simulink model "Assignment2"  (R2020a)
settings: Solver=FixedStepAuto  StartTime=0.0  StopTime=10.0  FixedStep=1e-3  RelTol=1e-3  EnableMultiTasking=on
undefined symbols (not defined in the file or in its folder): D0, D1, D10, D11, D12, D13, D2, D3, D4, D5, D6, D7, D8, D9, PTA0, PTA1, PTA2, PTB23, PTB9, PTC16, PTC17, PTC2, PTC3, PTC4, PTD0, PTD1, PTD2, PTD3
libraries: frdmk64flib x18, etargetslib x5
settings Model: ExtModeTrigDuration=5  Creator=iceca  LastModifiedBy=iceca
settings OptimizationCC: EnhancedBackFolding=on  PassReuseOutputArgsAs=Individual arguments  ZeroExternalMemoryAtStartup=off  ZeroInternalMemoryAtStartup=off  MaxStackSize=64  OptimizeBlockOrder=speed  DifferentSizesBufferReuse=on  OptimizationCustomize=off  EfficientTunableParamExpr=on
settings DebuggingCC: ParameterTunabilityLossMsg=error
settings HardwareCC: ProdBitPerPointer=32  ProdBitPerSizeT=32  ProdBitPerPtrDiffT=32  ProdLargestAtomicInteger=Long  ProdLargestAtomicFloat=Double  ProdWordSize=32  ProdHWDeviceType=ARM Compatible->ARM Cortex
settings SFSimCC: MATLABDynamicMemAlloc=off
settings RTWCC: SystemTargetFile=ert.tlc  HardwareBoard=NXP FRDM-K64F  TemplateMakefile=ert_default_tmf  Toolchain=GNU Tools for ARM Embedded Processors
settings CodeAppCC: ForceParamTrailComments=on  IgnoreCustomStorageClasses=off  OperatorAnnotations=on  SimulinkDataObjDesc=on  SFDataObjDesc=on  InsertBlockDesc=on

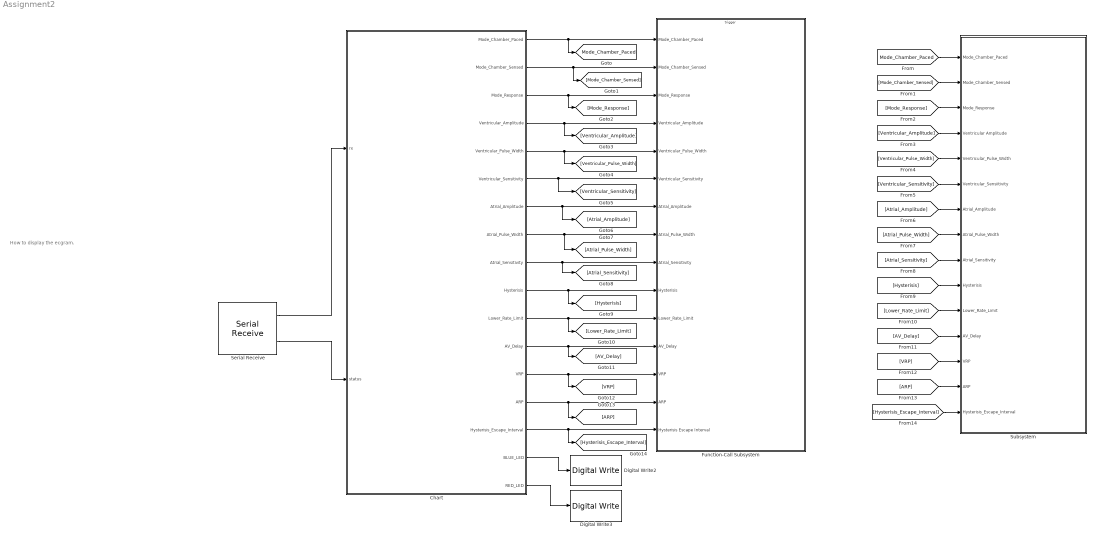
== system Assignment2 ==
  note: How to display the ecgram.
  Chart : Stateflow chart  TreatAsAtomicUnit=on
  Digital Write2 : frdmk64flib/Digital Write  Whichpin=BLUE_LED
  Digital Write3 : frdmk64flib/Digital Write  Whichpin=RED_LED
  Function-Call Subsystem : Subsystem  TreatAsAtomicUnit=on
  Serial Receive : frdmk64flib/Serial Receive  SCIModule=0  Baudrate=uint32(9600)  Parity=None  StopBits=1  HardwareFlowControl=None  ByteOrder=LittleEndian  DataType=uint8  DataLength=22  BlockingMode=off  OutputStatus=on  SampleTime=-1
  Subsystem : Subsystem
  tag scope: Mode_Chamber_Paced=global
  wires:
  Serial Receive/1 -> Chart/1(rx)
  Serial Receive/2 -> Chart/2(status)
  Chart/16(BLUE_LED) -> Digital Write2/1
  Chart/17(RED_LED) -> Digital Write3/1
  Chart/1(Mode_Chamber_Paced) -> [Mode_Chamber_Paced], Function-Call Subsystem/1(Mode_Chamber_Paced)
  Chart/10(Hysterisis) -> [Hysterisis], Function-Call Subsystem/10(Hysterisis)
  Chart/11(Lower_Rate_Limit) -> [Lower_Rate_Limit], Function-Call Subsystem/11(Lower_Rate_Limit)
  Chart/12(AV_Delay) -> [AV_Delay], Function-Call Subsystem/12(AV_Delay)
  Chart/13(VRP) -> [VRP], Function-Call Subsystem/13(VRP)
  Chart/14(ARP) -> [ARP], Function-Call Subsystem/14(ARP)
  Chart/15(Hysterisis_Escape_Interval) -> [Hysterisis_Escape_Interval], Function-Call Subsystem/15(Hysterisis Escape Interval)
  [Mode_Chamber_Paced] -> Subsystem/1(Mode_Chamber_Paced)
  Chart/2(Mode_Chamber_Sensed) -> [Mode_Chamber_Sensed], Function-Call Subsystem/2(Mode_Chamber_Sensed)
  Chart/3(Mode_Response) -> [Mode_Response], Function-Call Subsystem/3(Mode_Response)
  Chart/4(Ventricular_Amplitude) -> [Ventricular_Amplitude], Function-Call Subsystem/4(Ventricular_Amplitude)
  Chart/5(Ventricular_Pulse_Width) -> [Ventricular_Pulse_Width], Function-Call Subsystem/5(Ventricular_Pulse_Width)
  Chart/6(Ventricular_Sensitivity) -> [Ventricular_Sensitivity], Function-Call Subsystem/6(Ventricular_Sensitivity)
  Chart/7(Atrial_Amplitude) -> [Atrial_Amplitude], Function-Call Subsystem/7(Atrial_Amplitude)
  Chart/8(Atrial_Pulse_Width) -> [Atrial_Pulse_Width], Function-Call Subsystem/8(Atrial_Pulse_Width)
  Chart/9(Atrial_Sensitivity) -> [Atrial_Sensitivity], Function-Call Subsystem/9(Atrial_Sensitivity)
  [Mode_Chamber_Sensed] -> Subsystem/2(Mode_Chamber_Sensed)
  [Mode_Response] -> Subsystem/3(Mode_Response)
  [Ventricular_Amplitude] -> Subsystem/4(Ventricular Amplitude)
  [Ventricular_Pulse_Width] -> Subsystem/5(Ventricular_Pulse_Width)
  [Ventricular_Sensitivity] -> Subsystem/6(Ventricular_Sensiitivity)
  [Atrial_Amplitude] -> Subsystem/7(Atrial_Amplitude)
  [Atrial_Pulse_Width] -> Subsystem/8(Atrial_Pulse_Width)
  [Atrial_Sensitivity] -> Subsystem/9(Atrial_Sensitivity)
  [Hysterisis] -> Subsystem/10(Hysterisis)
  [Lower_Rate_Limit] -> Subsystem/11(Lower_Rate_Limit)
  [AV_Delay] -> Subsystem/12(AV_Delay)
  [VRP] -> Subsystem/13(VRP)
  [ARP] -> Subsystem/14(ARP)
  [Hysterisis_Escape_Interval] -> Subsystem/15(Hysterisis_Escape_Interval)

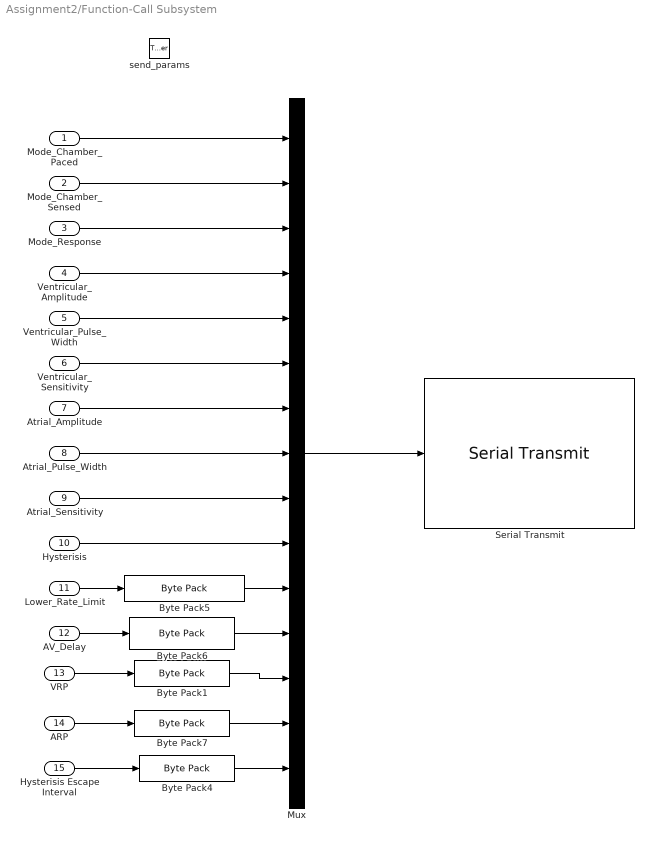
== system Assignment2/Function-Call Subsystem ==
  Mode_Chamber_Paced : Inport
  Mode_Chamber_Sensed : Inport  Port=2
  Mode_Response : Inport  Port=3
  Ventricular_Amplitude : Inport  Port=4
  Ventricular_Pulse_Width : Inport  Port=5
  Ventricular_Sensitivity : Inport  Port=6
  Atrial_Amplitude : Inport  Port=7
  Atrial_Pulse_Width : Inport  Port=8
  Atrial_Sensitivity : Inport  Port=9
  Hysterisis : Inport  Port=10
  Lower_Rate_Limit : Inport  Port=11
  AV_Delay : Inport  Port=12
  VRP : Inport  Port=13
  ARP : Inport  Port=14
  Hysterisis Escape Interval : Inport  Port=15
  send_params : TriggerPort  TriggerType=function-call  IsSimulinkFunction=on  FunctionName=send_params  VariantControl=Variant
  Byte Pack{1,4..7} (5 alike) : etargetslib/Byte Pack  datatypes={'uint16'}  byteAlign=1
  Mux : Mux  Inputs=15
  Serial Transmit : frdmk64flib/Serial Transmit  SCIModule=0  Baudrate=uint32(9600)  Parity=None  StopBits=1  HardwareFlowControl=None  ByteOrder=LittleEndian  BlockingMode=on  OutputStatus=off
  wires:
  Mode_Chamber_Paced/1 -> Mux/1
  Hysterisis/1 -> Mux/10
  Atrial_Pulse_Width/1 -> Mux/8
  Atrial_Amplitude/1 -> Mux/7
  Ventricular_Sensitivity/1 -> Mux/6
  Mode_Response/1 -> Mux/3
  Mode_Chamber_Sensed/1 -> Mux/2
  Atrial_Sensitivity/1 -> Mux/9
  Byte Pack1/1 -> Mux/13
  VRP/1 -> Byte Pack1/1
  Mux/1 -> Serial Transmit/1
  Ventricular_Amplitude/1 -> Mux/4
  Ventricular_Pulse_Width/1 -> Mux/5
  Hysterisis Escape Interval/1 -> Byte Pack4/1
  Lower_Rate_Limit/1 -> Byte Pack5/1
  AV_Delay/1 -> Byte Pack6/1
  Byte Pack6/1 -> Mux/12
  Byte Pack5/1 -> Mux/11
  Byte Pack7/1 -> Mux/14
  Byte Pack4/1 -> Mux/15
  ARP/1 -> Byte Pack7/1

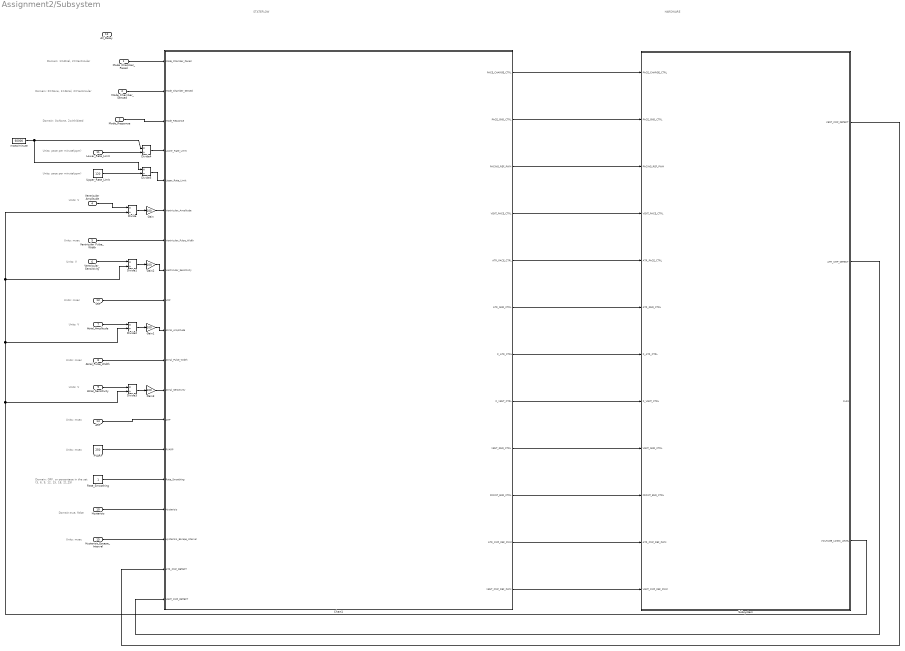
== system Assignment2/Subsystem ==
  note: Domain: OFF, or percentage
      | in the set (3, 6, 9, 12, 15, 18, 21,25)
  note: Domain: 0=None, 2=Inhibited
  note: Domain: 1=Atrial, 2=Ventricular
  note: Units: msec
  note: Units: pace per minute(ppm)
  note: HARDWARE
  note: Units: V
  note: STATEFLOW
  note: Units: msec
  note: Units: V
  note: Domain: 0=None, 1=Atrial, 2=Ventricular
  note: Units: pace per minute(ppm)
  note: Units: msec
  note: Units: msec
  note: Domain:true, false
  note: Units: V
  note: Units: msec
  note: Units: msec
  note: Units: V
  Mode_Chamber_Paced : Inport
  Mode_Chamber_Sensed : Inport  Port=2
  Mode_Response : Inport  Port=3
  Ventricular Amplitude : Inport  Port=4
  Ventricular_Pulse_Width : Inport  Port=5
  Ventricular_Sensiitivity : Inport  Port=6
  Atrial_Amplitude : Inport  Port=7
  Atrial_Pulse_Width : Inport  Port=8
  Atrial_Sensitivity : Inport  Port=9
  Hysterisis : Inport  Port=10
  Lower_Rate_Limit : Inport  Port=11
  AV_Delay : Inport  Port=12
  VRP : Inport  Port=13
  ARP : Inport  Port=14
  Hysterisis_Escape_Interval : Inport  Port=15
  Chart1 : Stateflow chart  TreatAsAtomicUnit=on
  Divide{,1..5} (6 alike) : Product  Inputs=*/
  Gain{,1..3} (4 alike) : Gain  Gain=100
  PVARP : Constant  Value=250
  Rate_Smoothing : Constant
  Subsystem : Subsystem
  Upper_Rate_Limit : Constant  Value=120
  msec/minute : Constant  Value=60000
  wires:
  Divide4/1 -> Chart1/4(Lower_Rate_Limit)
  Atrial_Pulse_Width/1 -> Chart1/11(Atrial_Pulse_Width)
  Atrial_Sensitivity/1 -> Divide3/1
  Divide/1 -> Gain/1
  Gain3/1 -> Chart1/12(Atrial_Sensitivity)
  PVARP/1 -> Chart1/14(PVARP)
  Gain/1 -> Chart1/6(Ventricular_Amplitude)
  Hysterisis/1 -> Chart1/16(Hysterisis)
  Ventricular Amplitude/1 -> Divide/1
  Chart1/8(Z_VENT_CTRL) -> Subsystem/8(Z_VENT_CTRL)
  Lower_Rate_Limit/1 -> Divide4/2
  Divide3/1 -> Gain3/1
  Subsystem/1(VENT_CMP_DETECT) -> Chart1/18(ATR_CMP_DETECT)
  Chart1/12(VENT_CMP_REF_PWM) -> Subsystem/12(VENT_CMP_REF_PWM)
  Divide2/1 -> Gain1/1
  Subsystem/2(ATR_CMP_DETECT) -> Chart1/19(VENT_CMP_DETECT)
  Hysterisis_Escape_Interval/1 -> Chart1/17(Hysterisis_Escape_Interval)
  Chart1/10(FRONT_END_CTRL) -> Subsystem/10(FRONT_END_CTRL)
  Chart1/7(Z_ATR_CTRL) -> Subsystem/7(Z_ATR_CTRL)
  Chart1/1(PACE_CHARGE_CTRL) -> Subsystem/1(PACE_CHARGE_CTRL)
  Rate_Smoothing/1 -> Chart1/15(Rate_Smoothing)
  Ventricular_Pulse_Width/1 -> Chart1/7(Ventricular_Pulse_Width)
  Ventricular_Sensiitivity/1 -> Divide1/1
  Chart1/11(ATR_CMP_REF_PWM) -> Subsystem/11(ATR_CMP_REF_PWM)
  Atrial_Amplitude/1 -> Divide2/1
  Chart1/6(ATR_GND_CTRL) -> Subsystem/6(ATR_GND_CTRL)
  Chart1/3(PACING_REF_PWM) -> Subsystem/3(PACING_REF_PWM)
  msec/minute/1 -> Divide5/1, Divide4/1
  Upper_Rate_Limit/1 -> Divide5/2
  Gain1/1 -> Chart1/10(Atrial_Amplitude)
  Chart1/2(PACE_GND_CTRL) -> Subsystem/2(PACE_GND_CTRL)
  Chart1/9(VENT_GND_CTRL) -> Subsystem/9(VENT_GND_CTRL)
  Chart1/4(VENT_PACE_CTRL) -> Subsystem/4(VENT_PACE_CTRL)
  VRP/1 -> Chart1/9(VRP)
  Divide5/1 -> Chart1/5(Upper_Rate_Limit)
  Chart1/5(ATR_PACE_CTRL) -> Subsystem/5(ATR_PACE_CTRL)
  Divide1/1 -> Gain2/1
  Gain2/1 -> Chart1/8(Ventricular_Sensitivity)
  Subsystem/4(VOLTAGE_LOGIC_LEVEL) -> Divide3/2, Divide2/2, Divide1/2, Divide/2
  Mode_Chamber_Paced/1 -> Chart1/1(Mode_Chamber_Paced)
  Mode_Chamber_Sensed/1 -> Chart1/2(Mode_Chamber_Sensed)
  Mode_Response/1 -> Chart1/3(Mode_Response)
  ARP/1 -> Chart1/13(ARP)

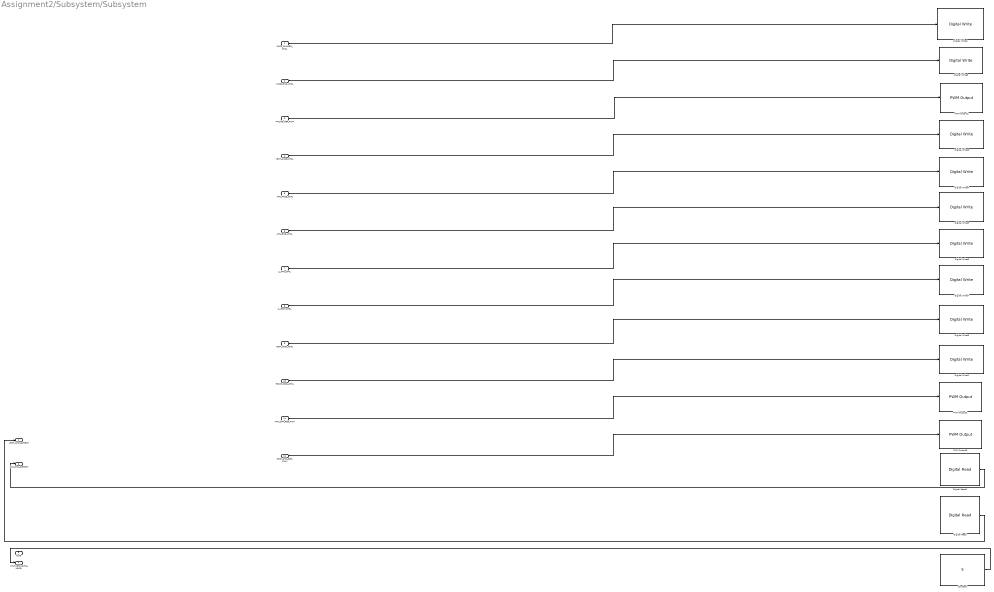
== system Assignment2/Subsystem/Subsystem ==
  PACE_CHARGE_CTRL : Inport
  PACE_GND_CTRL : Inport  Port=2
  PACING_REF_PWM : Inport  Port=3
  VENT_PACE_CTRL : Inport  Port=4
  ATR_PACE_CTRL : Inport  Port=5
  ATR_GND_CTRL : Inport  Port=6
  Z_ATR_CTRL : Inport  Port=7
  Z_VENT_CTRL : Inport  Port=8
  VENT_GND_CTRL : Inport  Port=9
  FRONT_END_CTRL : Inport  Port=10
  ATR_CMP_REF_PWM : Inport  Port=11
  VENT_CMP_REF_PWM : Inport  Port=12
  Constant : Constant  Value=5
  Digital Read : frdmk64flib/Digital Read  Whichpin=PTC16 (D0)  SampleTime=-1
  Digital Read1 : frdmk64flib/Digital Read  Whichpin=PTC17 (D1)  SampleTime=-1
  Digital Write1 : frdmk64flib/Digital Write  Whichpin=PTD1 (D13)
  Digital Write2 : frdmk64flib/Digital Write  Whichpin=PTB9 (D2)
  Digital Write3 : frdmk64flib/Digital Write  Whichpin=PTD0 (D10)
  Digital Write4 : frdmk64flib/Digital Write  Whichpin=PTA0 (D8)
  Digital Write5 : frdmk64flib/Digital Write  Whichpin=PTD2 (D11)
  Digital Write6 : frdmk64flib/Digital Write  Whichpin=PTB23 (D4)
  Digital Write7 : frdmk64flib/Digital Write  Whichpin=PTC3 (D7)
  Digital Write8 : frdmk64flib/Digital Write  Whichpin=PTC4 (D9)
  Digital Write9 : frdmk64flib/Digital Write  Whichpin=PTD3 (D12)
  PWM Output1 : frdmk64flib/PWM Output  Whichpin=PTA2 (D5)  InitialFrequency=2000  InitialDutyCycle=0
  PWM Output2 : frdmk64flib/PWM Output  Whichpin=PTC2 (D6)  InitialFrequency=2000  InitialDutyCycle=0
  PWM Output3 : frdmk64flib/PWM Output  Whichpin=PTA1 (D3)  InitialFrequency=2000  InitialDutyCycle=0
  VENT_CMP_DETECT : Outport
  ATR_CMP_DETECT : Outport  Port=2
  Out3 : Outport  Port=3
  VOLTAGE_LOGIC_LEVEL : Outport  Port=4
  wires:
  PACING_REF_PWM/1 -> PWM Output1/1
  VENT_GND_CTRL/1 -> Digital Write9/1
  PACE_GND_CTRL/1 -> Digital Write3/1
  ATR_GND_CTRL/1 -> Digital Write5/1
  ATR_CMP_REF_PWM/1 -> PWM Output2/1
  VENT_PACE_CTRL/1 -> Digital Write8/1
  Digital Read1/1 -> ATR_CMP_DETECT/1
  Digital Read/1 -> VENT_CMP_DETECT/1
  VENT_CMP_REF_PWM/1 -> PWM Output3/1
  Z_VENT_CTRL/1 -> Digital Write7/1
  Z_ATR_CTRL/1 -> Digital Write6/1
  PACE_CHARGE_CTRL/1 -> Digital Write2/1
  ATR_PACE_CTRL/1 -> Digital Write4/1
  FRONT_END_CTRL/1 -> Digital Write1/1
  Constant/1 -> VOLTAGE_LOGIC_LEVEL/1

== stateflow chart Assignment2/Subsystem/Chart1 ==
  note: |
  note: |
  note: 3 Sections: Atrial only States | Common States | Ventricular only States
  note: |
  note: |
  state Charging_C22
    entry:
    ATR_PACE_CTRL   = LOW;
    VENT_PACE_CTRL = LOW;
  note: Phase 1:
      | Charging Capacitors
  state Atrial_Charge
    entry:
    PACING_REF_PWM = Atrial_Amplitude;
  state Ventricular_Charge
    entry:
    PACING_REF_PWM = Ventricular_Amplitude;
  note: ----------------------------------------------------------------------------------
  state Discharging_C21_and_Pace_Interval_Calculations
    entry:
    PACE_CHARGE_CTRL = HIGH;
    %Discharging C21
    PACE_GND_CTRL=HIGH;
    VENT_PACE_CTRL=LOW;
    Z_ATR_CTRL= LOW;
    Z_VENT_CTRL = LOW;
    ATR_PACE_CTRL = LOW;
    Pace_Interval = Lower_Rate_Limit;
    if Hysterisis == HIGH
    Pace_Interval = Pace_Interval + Hysterisis_Escape_Interval;
    end
  note: Phase 2:
      | Discharging Capacitors
  state Atrial_Discharge
    entry:
    ATR_GND_CTRL= HIGH;
    VENT_GND_CTRL= LOW;
    Pace_Interval =Pace_Interval-Atrial_Pulse_Width;
  state Ventricular_Discharge
    entry:
    ATR_GND_CTRL = LOW;
    VENT_GND_CTRL = HIGH;
    Pace_Interval =Pace_Interval -Ventricular_Pulse_Width;
  note: ---------------------------------------------------------------------------------
  state Atrial_Sensing
    entry:
    FRONT_END_CTRL = HIGH;
    ATR_CMP_REF_PWM= Atrial_Sensitivity;
  state Ventricular_Sensing
    entry:
    FRONT_END_CTRL = HIGH;
    VENT_CMP_REF_PWM = Ventricular_Sensitivity;
  note: Phase 3:
      | Sensing
  state No_Natural_Activity_Sensed
  note: ----------------------------------------------------------------------------------
  state Pacing_Begin
    entry:
    PACE_CHARGE_CTRL = LOW;
    PACE_GND_CTRL = HIGH;
  note: Phase 4:
      | Pacing
  state Ventricular_Pacing
    entry:
    ATR_PACE_CTRL = LOW;
  state Atrial_Pacing
    entry:
    VENT_PACE_CTRL = LOW;
  state Pacing
    entry:
    ATR_GND_CTRL =LOW;
    Z_ATR_CTRL = LOW;
    Z_VENT_CTRL = LOW;
    VENT_GND_CTRL = LOW;
  state Vent_Pacing_2
    entry:
    VENT_PACE_CTRL =HIGH;
  state Atrial_Pacing_2
    entry:
    ATR_PACE_CTRL =HIGH;
  Vent_Pacing_2 -> Charging_C22 : [after(Ventricular_Pulse_Width,msec)]
  Atrial_Pacing_2 -> Charging_C22 : [after(Atrial_Pulse_Width,msec)]
  Ventricular_Sensing -> Charging_C22 [order 2] : [Mode_Response==2 &&  VENT_CMP_DETECT==true && after(VRP, msec)]
  Atrial_Sensing -> Charging_C22 [order 2] : [Mode_Response==2 && after(ARP, msec) && ATR_CMP_DETECT==HIGH]
  (default) -> Charging_C22
  Charging_C22 -> Atrial_Charge [order 2] : [Mode_Chamber_Paced==1]
  Charging_C22 -> Ventricular_Charge [order 1] : [Mode_Chamber_Paced==2]
  Atrial_Charge -> Discharging_C21_and_Pace_Interval_Calculations
  Ventricular_Charge -> Discharging_C21_and_Pace_Interval_Calculations
  Discharging_C21_and_Pace_Interval_Calculations -> Ventricular_Discharge [order 2] : [Mode_Chamber_Paced==2]
  Discharging_C21_and_Pace_Interval_Calculations -> Atrial_Discharge [order 1] : [Mode_Chamber_Paced==1]
  Atrial_Discharge -> Atrial_Sensing [order 2] : [Mode_Chamber_Sensed==1]
  Atrial_Discharge -> No_Natural_Activity_Sensed [order 1] : [Mode_Chamber_Sensed==0 && after(Pace_Interval, msec)]
  Ventricular_Discharge -> No_Natural_Activity_Sensed [order 2] : [Mode_Chamber_Sensed==0 && after(Pace_Interval, msec)]
  Ventricular_Discharge -> Ventricular_Sensing [order 1] : [Mode_Chamber_Sensed==2]
  Atrial_Sensing -> No_Natural_Activity_Sensed [order 1] : [after(Pace_Interval,msec)]
  Ventricular_Sensing -> No_Natural_Activity_Sensed [order 1] : [after(Pace_Interval,msec)]
  No_Natural_Activity_Sensed -> Pacing_Begin
  Pacing_Begin -> Ventricular_Pacing [order 1] : [Mode_Chamber_Paced==2]
  Pacing_Begin -> Atrial_Pacing [order 2] : [Mode_Chamber_Paced==1]
  Atrial_Pacing -> Pacing
  Ventricular_Pacing -> Pacing
  Pacing -> Atrial_Pacing_2 [order 2] : [Mode_Chamber_Paced==1]
  Pacing -> Vent_Pacing_2 [order 1] : [Mode_Chamber_Paced==2]
  data: Mode_Chamber_Paced input; Mode_Chamber_Sensed input; Mode_Response input; PACE_CHARGE_CTRL output; PACE_GND_CTRL output; PACING_REF_PWM output; VENT_PACE_CTRL output; ATR_PACE_CTRL output; ATR_GND_CTRL output; Z_ATR_CTRL output; Z_VENT_CTRL output; VENT_GND_CTRL output; Lower_Rate_Limit input; Upper_Rate_Limit input; HIGH local boolean =true; LOW local boolean =false; Ventricular_Amplitude input; Ventricular_Pulse_Width input; Ventricular_Sensitivity input; VRP input; Atrial_Amplitude input; Atrial_Pulse_Width input; Atrial_Sensitivity input; ARP input; PVARP input; Rate_Smoothing input; FRONT_END_CTRL output; ATR_CMP_REF_PWM output; VENT_CMP_REF_PWM output; Hysterisis input; Hysterisis_Escape_Interval input; ATR_CMP_DETECT input; VENT_CMP_DETECT input; Pace_Interval local

== stateflow chart Assignment2/Chart ==
  state SET_PARAMS
    entry:
    offset=3;
    RED_LED = true;
    %MODE
    Mode_Chamber_Paced=rx(offset);
    offset=offset+uint8_bytes;
    Mode_Chamber_Sensed=rx(offset);
    offset=offset+uint8_bytes;
    Mode_Response=rx(offset);
    offset=offset+uint8_bytes;
    %VENTRICLULAR PACE PARAMS
    Ventricular_Amplitude=rx(offset);
    offset=offset+uint8_bytes;
    Ventricular_Pulse_Width=rx(offset);
    offset=offset+uint8_bytes;
    Ventricular_Sensitivity=rx(offset);
    offset=offset+uint8_bytes;
    %ATRIAL PACE PARAMS
    Atrial_Amplitude=rx(offset);
    offset=offset+uint8_bytes;
    Atrial_Pulse_Width=rx(offset);
    offset=offset+uint8_bytes;
    Atrial_Sensitivity=rx(offset);
    offset=offset+uint8_bytes;
    %HYSTERISIS
    Hysterisis=rx(offset);
    offset=offset+uint8_bytes;
    %uint16 PARAMETERS
    Lower_Rate_Limit=typecast(rx(offset:offset+1),'uint16');
    offset=offset+uint16_bytes;
    AV_Delay=typecast(rx(offset:offset+1),'uint16');
    offset=offset+uint16_bytes;
    VRP=typecast(rx(offset:offset+1),'uint16');
    offset=offset+uint16_bytes;
    ARP=typecast(rx(offset:offset+1),'uint16');
    offset=offset+uint16_bytes;
    Hysterisis_Escape_Interval=typecast(rx(offset:offset+1),'uint16');
    offset=offset+uint16_bytes;
  note: TEST_CODE: 10
      | SET_CODE: 20
      | ECHO_CODEl 30
  state START_STATE
    entry:
    uint16_bytes = 2;
    uint8_bytes = 1;
  state WAIT_STATE
    entry:
    RED_LED=false;
    BLUE_LED=false;
  state ECHO_PARAMS
    entry:
    BLUE_LED = true;
    send_params();
  SET_PARAMS -> WAIT_STATE
  (junction 128) -> SET_PARAMS [order 1] : [rx(2) == 20]
  (default) -> START_STATE
  START_STATE -> WAIT_STATE
  (junction 132) -> WAIT_STATE [order 2]
  WAIT_STATE -> (junction 132) : [status == 0]
  (junction 132) -> (junction 128) [order 1] : [rx(1) == 10]
  (junction 128) -> ECHO_PARAMS [order 2] : [rx(2) == 30]
  ECHO_PARAMS -> WAIT_STATE
  data: Mode_Chamber_Paced output; Mode_Chamber_Sensed output; Mode_Response output; Ventricular_Amplitude output; Ventricular_Pulse_Width output; Ventricular_Sensitivity output; Atrial_Amplitude output; rx input uint8; offset local; Atrial_Pulse_Width output; Atrial_Sensitivity output; Hysterisis output; Lower_Rate_Limit output; AV_Delay output; VRP output; ARP output; Hysterisis_Escape_Interval output; status input uint8; uint16_bytes local; uint8_bytes local; BLUE_LED output; RED_LED output
